simulink model "gazebo_cosimulation_ideal_swarm_two"  (R2023b)
settings: Solver=VariableStepAuto  StartTime=0.0  StopTime=10.0  RelTol=1e-3
undefined symbols (not defined in the file): autonomous_quadcopter, center_cylinder, controlled_quadcopter, rotor_1, rotor_2, rotor_3, rotor_4
libraries: robotgazebolib x21, simulink x2
settings Model: Creator=rakshan  LastModifiedBy=rakshan

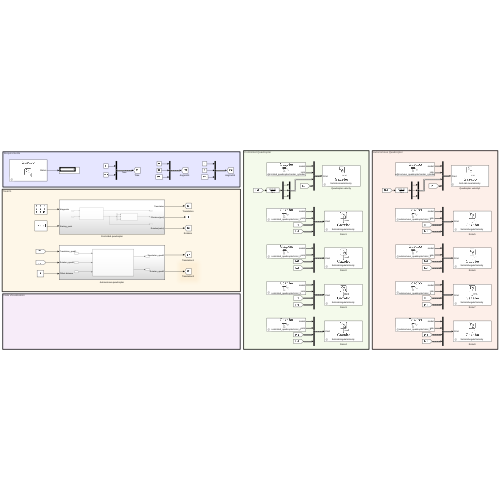
[thumbnail: Simulink's stored preview of the top-level diagram]
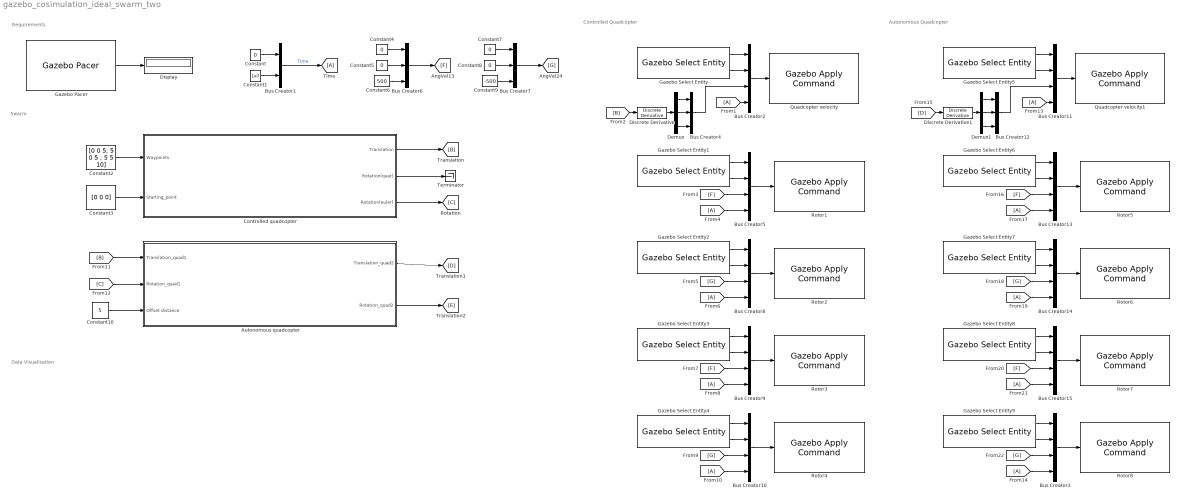
== system gazebo_cosimulation_ideal_swarm_two ==
  note: Requirements
  note: Data Visualisation
  note: Controlled Quadcopter
  note: Swarm
  note: Autonomous Quadcopter
  Autonomous quadcopter : Subsystem
  Bus Creator1 : BusCreator  Inputs=2  OutDataTypeStr=Bus: Gazebo_SL_Bus_gazebo_msgs_Time  NonVirtualBus=on
      settings: InheritFromInputs=off
  Bus Creator{3,5,8..10,13..15} (8 alike) : BusCreator  Inputs=4  OutDataTypeStr=Bus: Gazebo_SL_Bus_gazebo_msgs_SetLinkAngularVelocity  NonVirtualBus=on
      settings: InheritFromInputs=off
  Bus Creator11 : BusCreator  Inputs=4  OutDataTypeStr=Bus: Gazebo_SL_Bus_gazebo_msgs_SetLinkLinearVelocity  NonVirtualBus=on
      settings: InheritFromInputs=off
  Bus Creator{4,6..7,12} (4 alike) : BusCreator  Inputs=3  OutDataTypeStr=Bus: Gazebo_SL_Bus_gazebo_msgs_Point  NonVirtualBus=on
      settings: InheritFromInputs=off
  Bus Creator2 : BusCreator  Inputs=4  OutDataTypeStr=Bus: Gazebo_SL_Bus_gazebo_msgs_SetLinkLinearVelocity  NonVirtualBus=on
      settings: InheritFromInputs=off
  Constant{,4..5,7..8} (5 alike) : Constant  Value=0
  Constant1 : Constant  Value=1e7
  Constant10 : Constant  Value=5
  Constant2 : Constant  Value=[0 0 5; 5 0 5 ; 5 5 10]
  Constant3 : Constant  Value=[0 0 0]  VectorParams1D=off
  Constant6 : Constant  Value=500
  Constant9 : Constant  Value=-500
  Controlled quadcopter : Subsystem
  Demux : Demux  Outputs=3
  Demux1 : Demux  Outputs=3
  Discrete Derivative : simulink/Discrete/Discrete Derivative  gainval=1.0  ICPrevScaledInput=0.0  OutMin=[]  OutMax=[]  OutDataType=fixdt(1, 16)  OutScaling=2^-10  DoSatur=off
  Discrete Derivative1 : simulink/Discrete/Discrete Derivative  gainval=1.0  ICPrevScaledInput=0.0  OutMin=[]  OutMax=[]  OutDataType=fixdt(1, 16)  OutScaling=2^-10  DoSatur=off
  Display : Display
  From{1,4,6,8,10,13..14,17,19,21} (10 alike) : From
  Gazebo Pacer : robotgazebolib/Gazebo Pacer  ResetBehavior=Reset Gazebo simulation time  SampleTime=0.001
  Gazebo Select Entity : robotgazebolib/Gazebo Select Entity  modelElemName=controlled_quadcopter/center_cylinder  outputArraySize=128  OutputLabel=Link  SelectType=Link
  Gazebo Select Entity1 : robotgazebolib/Gazebo Select Entity  modelElemName=controlled_quadcopter/rotor_1  outputArraySize=128  OutputLabel=Link  SelectType=Link
  Gazebo Select Entity2 : robotgazebolib/Gazebo Select Entity  modelElemName=controlled_quadcopter/rotor_2  outputArraySize=128  OutputLabel=Link  SelectType=Link
  Gazebo Select Entity3 : robotgazebolib/Gazebo Select Entity  modelElemName=controlled_quadcopter/rotor_3  outputArraySize=128  OutputLabel=Link  SelectType=Link
  Gazebo Select Entity4 : robotgazebolib/Gazebo Select Entity  modelElemName=controlled_quadcopter/rotor_4  outputArraySize=128  OutputLabel=Link  SelectType=Link
  Gazebo Select Entity5 : robotgazebolib/Gazebo Select Entity  modelElemName=autonomous_quadcopter/center_cylinder  outputArraySize=128  OutputLabel=Link  SelectType=Link
  Gazebo Select Entity6 : robotgazebolib/Gazebo Select Entity  modelElemName=autonomous_quadcopter/rotor_1  outputArraySize=128  OutputLabel=Link  SelectType=Link
  Gazebo Select Entity7 : robotgazebolib/Gazebo Select Entity  modelElemName=autonomous_quadcopter/rotor_2  outputArraySize=128  OutputLabel=Link  SelectType=Link
  Gazebo Select Entity8 : robotgazebolib/Gazebo Select Entity  modelElemName=autonomous_quadcopter/rotor_3  outputArraySize=128  OutputLabel=Link  SelectType=Link
  Gazebo Select Entity9 : robotgazebolib/Gazebo Select Entity  modelElemName=autonomous_quadcopter/rotor_4  outputArraySize=128  OutputLabel=Link  SelectType=Link
  Quadcopter velocity : robotgazebolib/Gazebo Apply Command  cmdType=SetLinkLinearVelocity  sampleTime=0.001
  Quadcopter velocity1 : robotgazebolib/Gazebo Apply Command  cmdType=SetLinkLinearVelocity  sampleTime=0.001
  Rotor{1..8} (8 alike) : robotgazebolib/Gazebo Apply Command  cmdType=SetLinkAngularVelocity  sampleTime=0.001
  Terminator : Terminator
  Time : Goto
  wires:
  Gazebo Select Entity2/1 -> Bus Creator8/1
  Bus Creator2/1 -> Quadcopter velocity/1
  From8/1 -> Bus Creator9/4
  Gazebo Select Entity3/1 -> Bus Creator9/1
  From6/1 -> Bus Creator8/4
  Bus Creator7/1 -> [G]
  Gazebo Select Entity1/2 -> Bus Creator5/2
  Constant/1 -> Bus Creator1/1
  Gazebo Select Entity1/1 -> Bus Creator5/1
  Bus Creator1/1 -> Time/1  "Time"
  [F] -> Bus Creator5/3
  [G] -> Bus Creator10/3
  Gazebo Select Entity2/2 -> Bus Creator8/2
  Gazebo Select Entity4/1 -> Bus Creator10/1
  Bus Creator6/1 -> [F]
  Constant4/1 -> Bus Creator6/1
  Gazebo Select Entity3/2 -> Bus Creator9/2
  Bus Creator10/1 -> Rotor4/1
  [B] -> Discrete Derivative/1
  Constant6/1 -> Bus Creator6/3
  Demux/3 -> Bus Creator4/3
  From4/1 -> Bus Creator5/4
  [F] -> Bus Creator9/3
  Gazebo Select Entity/1 -> Bus Creator2/1
  Bus Creator4/1 -> Bus Creator2/3
  Constant9/1 -> Bus Creator7/3
  Gazebo Pacer/1 -> Display/1
  Constant1/1 -> Bus Creator1/2
  Bus Creator8/1 -> Rotor2/1
  Gazebo Select Entity/2 -> Bus Creator2/2
  From1/1 -> Bus Creator2/4
  Demux/2 -> Bus Creator4/2
  Bus Creator9/1 -> Rotor3/1
  Gazebo Select Entity4/2 -> Bus Creator10/2
  [G] -> Bus Creator8/3
  Discrete Derivative/1 -> Demux/1
  Constant7/1 -> Bus Creator7/1
  Constant8/1 -> Bus Creator7/2
  Bus Creator5/1 -> Rotor1/1
  Constant5/1 -> Bus Creator6/2
  Demux/1 -> Bus Creator4/1
  From10/1 -> Bus Creator10/4
  Constant3/1 -> Controlled quadcopter/2(Starting_point)
  Constant2/1 -> Controlled quadcopter/1(Waypoints)
  Controlled quadcopter/1(Translation) -> [B]
  Controlled quadcopter/2(Rotation(quat)) -> Terminator/1
  Controlled quadcopter/3(Rotation(euler)) -> [C]
  Autonomous quadcopter/1(Translation_quad2) -> [D]
  Autonomous quadcopter/2(Rotation_quad2) -> [E]
  [B] -> Autonomous quadcopter/1(Translation_quad1)
  [C] -> Autonomous quadcopter/2(Rotation_quad1)
  Constant10/1 -> Autonomous quadcopter/3(Offset distance)
  Bus Creator13/1 -> Rotor5/1
  Demux1/1 -> Bus Creator12/1
  From21/1 -> Bus Creator15/4
  Gazebo Select Entity5/2 -> Bus Creator11/2
  Gazebo Select Entity8/2 -> Bus Creator15/2
  Bus Creator14/1 -> Rotor6/1
  Gazebo Select Entity6/1 -> Bus Creator13/1
  Discrete Derivative1/1 -> Demux1/1
  Bus Creator12/1 -> Bus Creator11/3
  [F] -> Bus Creator15/3
  Gazebo Select Entity9/2 -> Bus Creator3/2
  Demux1/2 -> Bus Creator12/2
  Demux1/3 -> Bus Creator12/3
  [D] -> Discrete Derivative1/1
  From13/1 -> Bus Creator11/4
  Bus Creator3/1 -> Rotor8/1
  Gazebo Select Entity7/1 -> Bus Creator14/1
  Gazebo Select Entity8/1 -> Bus Creator15/1
  Gazebo Select Entity5/1 -> Bus Creator11/1
  [G] -> Bus Creator14/3
  [F] -> Bus Creator13/3
  Bus Creator11/1 -> Quadcopter velocity1/1
  Bus Creator15/1 -> Rotor7/1
  From17/1 -> Bus Creator13/4
  From19/1 -> Bus Creator14/4
  Gazebo Select Entity6/2 -> Bus Creator13/2
  [G] -> Bus Creator3/3
  Gazebo Select Entity7/2 -> Bus Creator14/2
  Gazebo Select Entity9/1 -> Bus Creator3/1
  From14/1 -> Bus Creator3/4

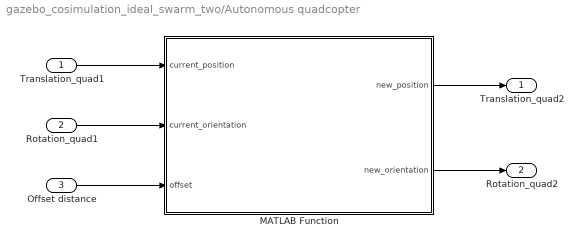
== system gazebo_cosimulation_ideal_swarm_two/Autonomous quadcopter ==
  Translation_quad1 : Inport
  Rotation_quad1 : Inport  Port=2
  Offset distance : Inport  Port=3
  MATLAB Function : MATLAB Function  TreatAsAtomicUnit=on
  Translation_quad2 : Outport
  Rotation_quad2 : Outport  Port=2
  wires:
  Rotation_quad1/1 -> MATLAB Function/2(current_orientation)
  Translation_quad1/1 -> MATLAB Function/1(current_position)
  Offset distance/1 -> MATLAB Function/3(offset)
  MATLAB Function/1(new_position) -> Translation_quad2/1
  MATLAB Function/2(new_orientation) -> Rotation_quad2/1

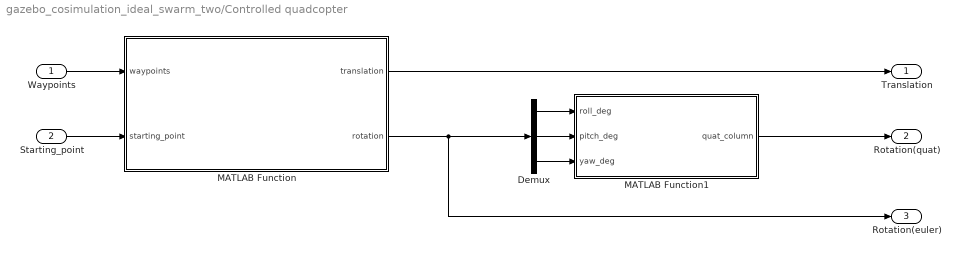
== system gazebo_cosimulation_ideal_swarm_two/Controlled quadcopter ==
  Waypoints : Inport
  Starting_point : Inport  Port=2
  Demux : Demux  Outputs=3
  MATLAB Function : MATLAB Function  TreatAsAtomicUnit=on
  MATLAB Function1 : MATLAB Function  TreatAsAtomicUnit=on
  Translation : Outport
  Rotation(quat) : Outport  Port=2
  Rotation(euler) : Outport  Port=3
  wires:
  Demux/1 -> MATLAB Function1/1(roll_deg)
  Demux/3 -> MATLAB Function1/3(yaw_deg)
  Demux/2 -> MATLAB Function1/2(pitch_deg)
  MATLAB Function1/1(quat_column) -> Rotation(quat)/1
  MATLAB Function/2(rotation) -> Rotation(euler)/1, Demux/1
  Waypoints/1 -> MATLAB Function/1(waypoints)
  Starting_point/1 -> MATLAB Function/2(starting_point)
  MATLAB Function/1(translation) -> Translation/1

== matlab function gazebo_cosimulation_ideal_swarm_two/Controlled quadcopter/MATLAB Function ==
  data: waypoints input; translation output; rotation output; starting_point input
function [translation, rotation] = interpolateWaypointsSimulink(waypoints,starting_point)
    persistent current_waypoint;
    persistent current_index;
    time_step = 0.002;
   
    waypoints = [starting_point;waypoints]
    % Initialize persistent variables on first call
    if isempty(current_waypoint)
        current_waypoint = waypoints(1,:);
        current_index = 1;
    end
    
    % Initialize outputs
    translation = zeros(1, 3);
    rotation = zeros(1, 3); % Euler angles: [yaw, pitch, roll]
    
    % Check if reached last waypoint
    if current_index == size(waypoints, 1)
        translation = waypoints(end, :);
        rotation = [0 0 0]; % No rotation (identity)
    else
        % Interpolate translation
        translation = current_waypoint;
        next_waypoint = waypoints(current_index + 1, :);
        current_waypoint = current_waypoint + (next_waypoint - current_waypoint) * time_step;
        
        % Calculate direction vector
        direction_vector = next_waypoint - current_waypoint;
        direction_vector = direction_vector / norm(direction_vector); % Normalize
        
        % Calculate rotation angles (Euler angles)
        yaw = atan2(direction_vector(2), direction_vector(1));
        pitch = asin(direction_vector(3));
        roll = 0; % Assuming no roll motion
        
        % Update rotation
        rotation = [yaw pitch roll];
        
        % Check if reached next waypoint
        if norm(current_waypoint - next_waypoint) < 0.01
            current_index = current_index + 1;
        end
    end
end

== matlab function gazebo_cosimulation_ideal_swarm_two/Autonomous quadcopter/MATLAB Function ==
  data: current_position input; new_position output; current_orientation input; offset input; new_orientation output
function [new_position, new_orientation] = addXOffsetFunction(current_position, current_orientation,offset)
    % Add the offset to the x position
    new_position = current_position;
    new_position(1) = new_position(1) + offset;

    % Orientation remains the same
    new_orientation = current_orientation;
end

== matlab function gazebo_cosimulation_ideal_swarm_two/Controlled quadcopter/MATLAB Function1 ==
  data: roll_deg input; quat_column output; pitch_deg input; yaw_deg input
function quat_column = eulerToQuat(roll_deg, pitch_deg, yaw_deg)
    % Convert Euler angles to radians
    roll_rad = deg2rad(roll_deg);
    pitch_rad = deg2rad(pitch_deg);
    yaw_rad = deg2rad(yaw_deg);

    % Calculate half angles
    roll_half = roll_rad / 2;
    pitch_half = pitch_rad / 2;
    yaw_half = yaw_rad / 2;

    % Calculate trigonometric functions
    roll_sin = sin(roll_half);
    roll_cos = cos(roll_half);
    pitch_sin = sin(pitch_half);
    pitch_cos = cos(pitch_half);
    yaw_sin = sin(yaw_half);
    yaw_cos = cos(yaw_half);

    % Calculate quaternion components
    q0 = roll_cos * pitch_cos * yaw_cos + roll_sin * pitch_sin * yaw_sin;
    q1 = roll_sin * pitch_cos * yaw_cos - roll_cos * pitch_sin * yaw_sin;
    q2 = roll_cos * pitch_sin * yaw_cos + roll_sin * pitch_cos * yaw_sin;
    q3 = roll_cos * pitch_cos * yaw_sin - roll_sin * pitch_sin * yaw_cos;

    % Format the quaternion as a column vector
    quat_column = [q0; q1; q2; q3];
end
